simulink model "deney3-2"  (R2023b)
settings: Solver=VariableStepAuto  StartTime=0.0  StopTime=5  RelTol=1e-3
libraries: dspfdesign x1, commrandsrc3 x1, commutil2 x1
settings Model: Creator=Berkay Yalçın  LastModifiedBy=Berkay Yalçın

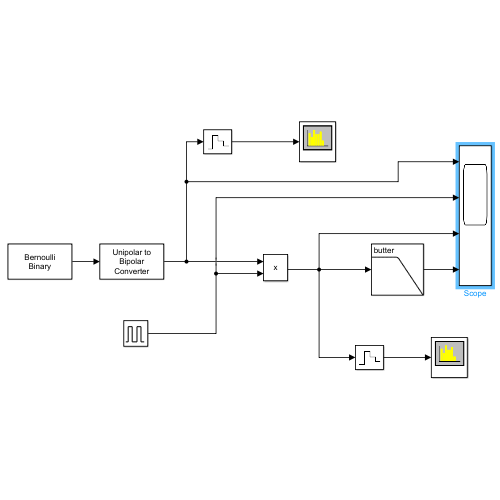
[thumbnail: Simulink's stored preview of the top-level diagram]
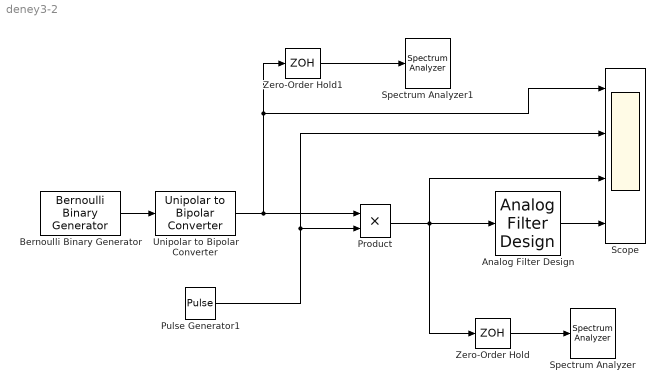
== system deney3-2 ==
  Analog Filter Design : dspfdesign/Analog Filter Design  method=Butterworth  filttype=Lowpass  N=8  Wlo=30  Whi=80  Rp=2  Rs=40
  Bernoulli Binary Generator : commrandsrc3/Bernoulli Binary Generator  ProbabilityOfZero=0.5  SeedSource=Auto  Seed=0  SampleTime=1/1000  SamplesPerFrame=1  OutputDataType=double  SimulateUsing=Code generation
  Product : Product
  Pulse Generator1 : DiscretePulseGenerator  PulseType=Time based  Amplitude=5  Period=1/1000  PulseWidth=75
  Scope : Scope  NumInputPorts=4
  Spectrum Analyzer : SpectrumAnalyzer  WindowPosition=[303.000000,149.000000,799.000000,500.000000,]  Visible=on  ScopeFrameLocation=window  Span=1000  StartFrequency=-500  StopFrequency=500  YLimits=[-78.97754909,-22.26479758]
  Spectrum Analyzer1 : SpectrumAnalyzer  WindowPosition=[1.000000,49.000000,1536.000000,793.000000,]  ScopeFrameLocation=window
  Unipolar to Bipolar Converter : commutil2/Unipolar to Bipolar Converter  M=2  polarity=Positive  dataType=Inherit via internal rule
  Zero-Order Hold : ZeroOrderHold  SampleTime=-1
  Zero-Order Hold1 : ZeroOrderHold  SampleTime=0.1
  wires:
  Bernoulli Binary Generator/1 -> Unipolar to Bipolar Converter/1
  Product/1 -> Scope/3, Analog Filter Design/1, Zero-Order Hold/1
  Pulse Generator1/1 -> Scope/2, Product/2
  Zero-Order Hold1/1 -> Spectrum Analyzer1/1
  Zero-Order Hold/1 -> Spectrum Analyzer/1
  Analog Filter Design/1 -> Scope/4
  Unipolar to Bipolar Converter/1 -> Zero-Order Hold1/1, Scope/1, Product/1
